simulink model "RUN_ME3_Helicopter_System_CDR"  (R2020b)
settings: Solver=VariableStepAuto  StartTime=0.0  StopTime=All_Sim_time  RelTol=1e-3
values from neighbouring files (symbols this model uses):
  All_Delay_betwn_actns = 28    [RUN_ME2_gui_to_tragectory.m]    (also in Workspace_CDR.mat = 30)
  All_Maneuver_smoothness = 16    [RUN_ME2_gui_to_tragectory.m]    (also in Workspace_CDR.mat = 28)
  K_CABLE = 3    [Coefficient_CDR.m]    (also in Workspace_CDR.mat)
  Kd_2 = PID_Elev_2.kd    [Coefficient_CDR.m]    (also in Workspace_CDR.mat = 79.7976366439)
  Kdp_2p = PID_Pitch_new_2pole.kd    [Coefficient_CDR.m]    (also in Workspace_CDR.mat = 43.0143282827)
  Kdt_2pole = PID_Travel_2pole.kd    [Coefficient_CDR.m]    (also in Workspace_CDR.mat = -1.1577862566)
  Ki_2 = PID_Elev_2.ki    [Coefficient_CDR.m]    (also in Workspace_CDR.mat = 88.2222308128)
  Kip_2p = PID_Pitch_new_2pole.ki    [Coefficient_CDR.m]    (also in Workspace_CDR.mat = 0)
  Kit_2pole = PID_Travel_2pole.ki    [Coefficient_CDR.m]    (also in Workspace_CDR.mat = -0.231061623642)
  Kp_2 = PID_Elev_2.kp    [Coefficient_CDR.m]    (also in Workspace_CDR.mat = 169.271716506)
  Kpp_2p = PID_Pitch_new_2pole.kp    [Coefficient_CDR.m]    (also in Workspace_CDR.mat = 367.16787657)
  Kpt_2pole = PID_Travel_2pole.kp    [Coefficient_CDR.m]    (also in Workspace_CDR.mat = -1.06540125736)
  Maneuver1_aggression = 20    [RUN_ME2_gui_to_tragectory.m]    (also in Workspace_CDR.mat)
  Maneuver2_aggression = 5    [RUN_ME2_gui_to_tragectory.m]    (also in Workspace_CDR.mat = 45)
  Maneuver3_aggression = 3    [RUN_ME2_gui_to_tragectory.m]    (also in Workspace_CDR.mat = 6.8)
  Maneuver4_aggression = 0.3    [RUN_ME2_gui_to_tragectory.m]    (also in Workspace_CDR.mat = 0.8)
  Maneuver5_aggression = 3.5    [RUN_ME2_gui_to_tragectory.m]    (also in Workspace_CDR.mat = 2.5)
libraries: simulink_extras x5, pid_lib x3, cstblocks x3
settings Model: Creator=justin  LastModifiedBy=liors

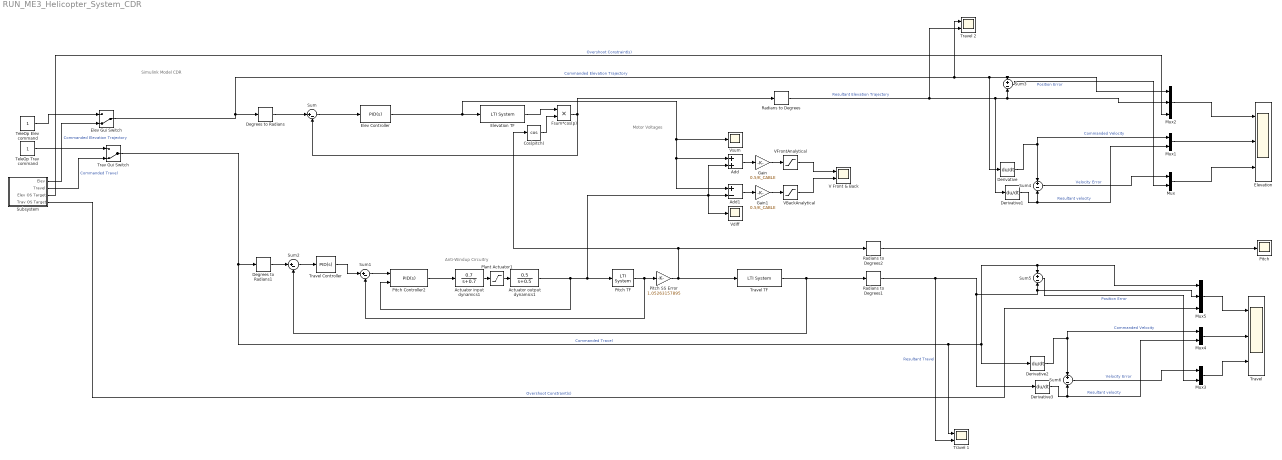
== system RUN_ME3_Helicopter_System_CDR ==
  note: Motor Voltages
  note: Anti-Windup Circuitry
  note: Simulink Model
      | CDR
  Actuator input dynamics1 : TransferFcn  Numerator=[0.7]  Denominator=[1 0.7]
  Actuator output dynamics1 : TransferFcn  Numerator=[0.5]  Denominator=[1 0.5]
  Add : Sum
  Add1 : Sum  Inputs=+-
  Cos(pitch) : Trigonometry  Operator=cos
  Degrees to Radians : simulink_extras/Transformations/Degrees to Radians
  Degrees to Radians1 : simulink_extras/Transformations/Degrees to Radians
  Derivative{,1..3} (4 alike) : Derivative
  Elev Controller : pid_lib/PID Controller  Controller=PID  Form=Parallel  TimeDomain=Continuous-time  UseExternalTs=off  SampleTime=-1  IntegratorMethod=Forward Euler  FilterMethod=Forward Euler  ControllerParametersSource=internal  P=Kp_2  I=Ki_2  D=Kd_2  UseFilter=on  N=100  TunerSelectOption=Transfer Function Based (PID Tuner App)  InitialConditionSource=internal  InitialConditionForIntegrator=0  InitialConditionForFilter=0  DifferentiatorICPrevScaledInput=0  ExternalReset=none  TrackingMode=off  Kt=150  LimitOutput=off  SatLimitsSource=internal  UpperSaturationLimit=inf  LowerSaturationLimit=0  LinearizeAsGain=on  AntiWindupMode=none  Kb=1  POutMin=[]  POutMax=[]  IOutMin=[]  IOutMax=[]  DOutMin=[]  DOutMax=[]  NOutMin=[]  NOutMax=[]  SumOutMin=[]  SumOutMax=[]  SaturationOutMin=[]  SaturationOutMax=[]  PParamMin=[]  PParamMax=[]  IParamMin=[]  IParamMax=[]  DParamMin=[]  DParamMax=[]  NParamMin=[]  NParamMax=[]  KbParamMin=[]  KbParamMax=[]  KtParamMin=[]  KtParamMax=[]  KbOutMin=[]  KbOutMax=[]  KtOutMin=[]  KtOutMax=[]  IntegratorOutMin=[]  IntegratorOutMax=[]  FilterOutMin=[]  FilterOutMax=[]  SumI1OutMin=[]  SumI1OutMax=[]  SumI2OutMin=[]  SumI2OutMax=[]  SumI3OutMin=[]  SumI3OutMax=[]  SumI4OutMin=[]  SumI4OutMax=[]  SumDOutMin=[]  SumDOutMax=[]  DifferentiatorOutMin=[]  DifferentiatorOutMax=[]  FilterDiffOutCoefMin=[]  FilterDiffOutCoefMax=[]  ReciprocalOutMin=[]  ReciprocalOutMax=[]  SumDenOutMin=[]  SumDenOutMax=[]  SumNumOutMin=[]  SumNumOutMax=[]  DivideOutMin=[]  DivideOutMax=[]  UdiffTsProdOutMin=[]  UdiffTsProdOutMax=[]  NTsProdOutMin=[]  NTsProdOutMax=[]  UintegralTsProdOutMin=[]  UintegralTsProdOutMax=[]  UngainTsProdOutMin=[]  UngainTsProdOutMax=[]  IntegratorContinuousStateAttributes=''  IntegratorStateMustResolveToSignalObject=off  IntegratorRTWStateStorageClass=Auto  FilterContinuousStateAttributes=''  FilterStateMustResolveToSignalObject=off  FilterRTWStateStorageClass=Auto  ParallelPVariant=InternalParameters  IdealPVariant=Disabled  IVariant=InternalParameters  DVariant=InternalParameters  IntegratorVariant=Continuous  SatVariant=Disabled  AWVariant=Passthrough  PCopyVariant=Disabled  TRVariant=Disabled  FdbkBlocksVariant=Forward  IdealPFdbkVariant=Disabled  SatFdbkVariant=Disabled  DerivativeFilterVariant=ContFilter  NVariant=InternalParameters  NCopyVariant=Disabled  FilterICVariant=InternalICsFilter  IntegratorICVariant=InternalICs  ExternalResetVariant=Disabled  TRSumVariant=Passthrough  SumFdbkVariant=Disabled  SumVariant=Sum_PID  TsampFilterVariant=InternalTs  TsampNgainVariant=Passthrough  TsampIntegralVariant=Passthrough  ExternalSaturationOutDataTypeStr=Inherit: Same as second input
  Elev Gui Switch : ManualSwitch  CurrentSetting=0
  Elevation : Scope  NumInputPorts=3
  Elevation TF : cstblocks/LTI System  sys=sys  IC=[-5.18]
  Fsum*cos(p) : Product
  Gain : Gain  Gain=0.5/K_CABLE
  Gain1 : Gain  Gain=0.5/K_CABLE
  Mux{,1,3..4} (4 alike) : Mux  Inputs=2
  Mux2 : Mux  Inputs=3
  Mux5 : Mux  Inputs=3
  "Pitch " : Scope
  Pitch Controller2 : pid_lib/PID Controller  Controller=PID  Form=Parallel  TimeDomain=Continuous-time  UseExternalTs=off  SampleTime=-1  IntegratorMethod=Forward Euler  FilterMethod=Forward Euler  ControllerParametersSource=internal  P=Kpp_2p  I=Kip_2p  D=Kdp_2p  UseFilter=on  N=100  TunerSelectOption=Transfer Function Based (PID Tuner App)  InitialConditionSource=internal  InitialConditionForIntegrator=0  InitialConditionForFilter=0  DifferentiatorICPrevScaledInput=0  ExternalReset=none  TrackingMode=on  Kt=75  LimitOutput=off  SatLimitsSource=internal  UpperSaturationLimit=2.94  LowerSaturationLimit=-2.94  LinearizeAsGain=on  AntiWindupMode=back-calculation  Kb=1000  POutMin=[]  POutMax=[]  IOutMin=[]  IOutMax=[]  DOutMin=[]  DOutMax=[]  NOutMin=[]  NOutMax=[]  SumOutMin=[]  SumOutMax=[]  SaturationOutMin=[]  SaturationOutMax=[]  PParamMin=[]  PParamMax=[]  IParamMin=[]  IParamMax=[]  DParamMin=[]  DParamMax=[]  NParamMin=[]  NParamMax=[]  KbParamMin=[]  KbParamMax=[]  KtParamMin=[]  KtParamMax=[]  KbOutMin=[]  KbOutMax=[]  KtOutMin=[]  KtOutMax=[]  IntegratorOutMin=[]  IntegratorOutMax=[]  FilterOutMin=[]  FilterOutMax=[]  SumI1OutMin=[]  SumI1OutMax=[]  SumI2OutMin=[]  SumI2OutMax=[]  SumI3OutMin=[]  SumI3OutMax=[]  SumI4OutMin=[]  SumI4OutMax=[]  SumDOutMin=[]  SumDOutMax=[]  DifferentiatorOutMin=[]  DifferentiatorOutMax=[]  FilterDiffOutCoefMin=[]  FilterDiffOutCoefMax=[]  ReciprocalOutMin=[]  ReciprocalOutMax=[]  SumDenOutMin=[]  SumDenOutMax=[]  SumNumOutMin=[]  SumNumOutMax=[]  DivideOutMin=[]  DivideOutMax=[]  UdiffTsProdOutMin=[]  UdiffTsProdOutMax=[]  NTsProdOutMin=[]  NTsProdOutMax=[]  UintegralTsProdOutMin=[]  UintegralTsProdOutMax=[]  UngainTsProdOutMin=[]  UngainTsProdOutMax=[]  IntegratorContinuousStateAttributes=''  IntegratorStateMustResolveToSignalObject=off  IntegratorRTWStateStorageClass=Auto  FilterContinuousStateAttributes=''  FilterStateMustResolveToSignalObject=off  FilterRTWStateStorageClass=Auto  ParallelPVariant=InternalParameters  IdealPVariant=Disabled  IVariant=InternalParameters  DVariant=InternalParameters  IntegratorVariant=Continuous  SatVariant=Disabled  AWVariant=Passthrough  PCopyVariant=Disabled  TRVariant=Enabled  FdbkBlocksVariant=Forward  IdealPFdbkVariant=Disabled  SatFdbkVariant=Disabled  DerivativeFilterVariant=ContFilter  NVariant=InternalParameters  NCopyVariant=Disabled  FilterICVariant=InternalICsFilter  IntegratorICVariant=InternalICs  ExternalResetVariant=Disabled  TRSumVariant=TrackingMode  SumFdbkVariant=Disabled  SumVariant=Sum_PID  TsampFilterVariant=InternalTs  TsampNgainVariant=Passthrough  TsampIntegralVariant=Passthrough  ExternalSaturationOutDataTypeStr=Inherit: Same as second input
  Pitch SS Error : Gain  Gain=1.05263157895
  Pitch TF : cstblocks/LTI System  sys=G_Pitch_new_2pole_1  IC=[]
  Plant Actuator1 : Saturate  UpperLimit=4  LowerLimit=-4
  Radians to Degrees : simulink_extras/Transformations/Radians to Degrees
  Radians to Degrees1 : simulink_extras/Transformations/Radians to Degrees
  Radians to Degrees2 : simulink_extras/Transformations/Radians to Degrees
  Subsystem : Subsystem
  Sum : Sum  Inputs=|+-
  Sum1 : Sum  Inputs=|+-
  Sum2 : Sum  Inputs=|+-
  Sum{3..6} (4 alike) : Sum  Inputs=+|-
  TeleOp Elev command : Constant
  TeleOp Trav command : Constant
  Trav Gui Switch : ManualSwitch  CurrentSetting=0
  Travel : Scope  NumInputPorts=3
  Travel 1 : Scope  NumInputPorts=2
  Travel 2 : Scope  NumInputPorts=2
  Travel Controller : pid_lib/PID Controller  Controller=PID  Form=Parallel  TimeDomain=Continuous-time  UseExternalTs=off  SampleTime=-1  IntegratorMethod=Forward Euler  FilterMethod=Forward Euler  ControllerParametersSource=internal  P=Kpt_2pole  I=Kit_2pole  D=Kdt_2pole  UseFilter=on  N=100  TunerSelectOption=Transfer Function Based (PID Tuner App)  InitialConditionSource=internal  InitialConditionForIntegrator=0  InitialConditionForFilter=0  DifferentiatorICPrevScaledInput=0  ExternalReset=none  TrackingMode=off  Kt=1  LimitOutput=off  SatLimitsSource=internal  UpperSaturationLimit=inf  LowerSaturationLimit=-inf  LinearizeAsGain=on  AntiWindupMode=none  Kb=1  POutMin=[]  POutMax=[]  IOutMin=[]  IOutMax=[]  DOutMin=[]  DOutMax=[]  NOutMin=[]  NOutMax=[]  SumOutMin=[]  SumOutMax=[]  SaturationOutMin=[]  SaturationOutMax=[]  PParamMin=[]  PParamMax=[]  IParamMin=[]  IParamMax=[]  DParamMin=[]  DParamMax=[]  NParamMin=[]  NParamMax=[]  KbParamMin=[]  KbParamMax=[]  KtParamMin=[]  KtParamMax=[]  KbOutMin=[]  KbOutMax=[]  KtOutMin=[]  KtOutMax=[]  IntegratorOutMin=[]  IntegratorOutMax=[]  FilterOutMin=[]  FilterOutMax=[]  SumI1OutMin=[]  SumI1OutMax=[]  SumI2OutMin=[]  SumI2OutMax=[]  SumI3OutMin=[]  SumI3OutMax=[]  SumI4OutMin=[]  SumI4OutMax=[]  SumDOutMin=[]  SumDOutMax=[]  DifferentiatorOutMin=[]  DifferentiatorOutMax=[]  FilterDiffOutCoefMin=[]  FilterDiffOutCoefMax=[]  ReciprocalOutMin=[]  ReciprocalOutMax=[]  SumDenOutMin=[]  SumDenOutMax=[]  SumNumOutMin=[]  SumNumOutMax=[]  DivideOutMin=[]  DivideOutMax=[]  UdiffTsProdOutMin=[]  UdiffTsProdOutMax=[]  NTsProdOutMin=[]  NTsProdOutMax=[]  UintegralTsProdOutMin=[]  UintegralTsProdOutMax=[]  UngainTsProdOutMin=[]  UngainTsProdOutMax=[]  IntegratorContinuousStateAttributes=''  IntegratorStateMustResolveToSignalObject=off  IntegratorRTWStateStorageClass=Auto  FilterContinuousStateAttributes=''  FilterStateMustResolveToSignalObject=off  FilterRTWStateStorageClass=Auto  ParallelPVariant=InternalParameters  IdealPVariant=Disabled  IVariant=InternalParameters  DVariant=InternalParameters  IntegratorVariant=Continuous  SatVariant=Disabled  AWVariant=Passthrough  PCopyVariant=Disabled  TRVariant=Disabled  FdbkBlocksVariant=Forward  IdealPFdbkVariant=Disabled  SatFdbkVariant=Disabled  DerivativeFilterVariant=ContFilter  NVariant=InternalParameters  NCopyVariant=Disabled  FilterICVariant=InternalICsFilter  IntegratorICVariant=InternalICs  ExternalResetVariant=Disabled  TRSumVariant=Passthrough  SumFdbkVariant=Disabled  SumVariant=Sum_PID  TsampFilterVariant=InternalTs  TsampNgainVariant=Passthrough  TsampIntegralVariant=Passthrough  ExternalSaturationOutDataTypeStr=Inherit: Same as second input
  Travel TF : cstblocks/LTI System  sys=G_Travel_new_2pole_1  IC=[]
  V Front & Back : Scope  NumInputPorts=2
  VBackAnalytical : Saturate  UpperLimit=22  LowerLimit=-22
  VFrontAnalytical : Saturate  UpperLimit=22  LowerLimit=-22
  Vdiff : Scope
  Vsum : Scope
  wires:
  Radians to Degrees/1 -> Travel 2/2, Mux2/2, Sum3/2, Derivative1/1  "Resultant Elevation Trajectory"
  Fsum*cos(p)/1 -> Sum/2, Radians to Degrees/1
  Travel TF/1 -> Sum2/2, Radians to Degrees1/1
  Degrees to Radians1/1 -> Sum2/1
  Radians to Degrees1/1 -> Travel 1/2, Derivative3/1, Mux5/2, Sum5/2  "Resultant Travel"
  Add/1 -> Gain/1
  Add1/1 -> Gain1/1
  Radians to Degrees2/1 -> "Pitch "/1
  Elev Gui Switch/1 -> Travel 2/1, Derivative/1, Sum3/1, Mux2/1, Degrees to Radians/1  "Commanded Elevation Trajectory"
  Gain/1 -> VFrontAnalytical/1
  VFrontAnalytical/1 -> V Front & Back/1
  Gain1/1 -> VBackAnalytical/1
  VBackAnalytical/1 -> V Front & Back/2
  Degrees to Radians/1 -> Sum/1
  Sum/1 -> Elev Controller/1
  Sum2/1 -> Travel Controller/1
  Cos(pitch)/1 -> Fsum*cos(p)/2
  Pitch TF/1 -> Pitch SS Error/1, Sum1/2
  Actuator input dynamics1/1 -> Plant Actuator1/1
  Plant Actuator1/1 -> Actuator output dynamics1/1
  Elev Controller/1 -> Add1/1, Add/1, Vsum/1, Elevation TF/1
  Actuator output dynamics1/1 -> Pitch Controller2/2, Vdiff/1, Add/2, Add1/2, Pitch TF/1
  Sum1/1 -> Pitch Controller2/1
  Travel Controller/1 -> Sum1/1
  Pitch SS Error/1 -> Cos(pitch)/1, Radians to Degrees2/1, Travel TF/1
  Pitch Controller2/1 -> Actuator input dynamics1/1
  Subsystem/3(Elev OS Target) -> Mux2/3  "Overshoot Constraint(s)"
  Subsystem/4(Trav OS Target) -> Mux5/3  "Overshoot Constraint(s)"
  Derivative/1 -> Mux1/1, Sum4/1  "Commanded Velocity"
  Derivative1/1 -> Sum4/2, Mux1/2  "Resultant velocity"
  Mux2/1 -> Elevation/1
  Mux1/1 -> Elevation/2
  Mux/1 -> Elevation/3
  Sum3/1 -> Mux/2  "Position Error"
  Sum4/1 -> Mux/1  "Velocity Error"
  Mux4/1 -> Travel/2
  Derivative2/1 -> Mux4/1, Sum6/1  "Commanded Velocity"
  Derivative3/1 -> Sum6/2, Mux4/2  "Resultant velocity"
  Sum5/1 -> Mux3/2  "Position Error"
  Mux5/1 -> Travel/1
  Mux3/1 -> Travel/3
  Sum6/1 -> Mux3/1  "Velocity Error"
  Trav Gui Switch/1 -> Travel 1/1, Mux5/1, Sum5/1, Derivative2/1, Degrees to Radians1/1  "Commanded Travel"
  TeleOp Trav command/1 -> Trav Gui Switch/1
  Subsystem/2(Travel) -> Trav Gui Switch/2  "Commanded Travel"
  Subsystem/1(Elev) -> Elev Gui Switch/2  "Commanded Elevation Trajectory"
  TeleOp Elev command/1 -> Elev Gui Switch/1
  Elevation TF/1 -> Fsum*cos(p)/1

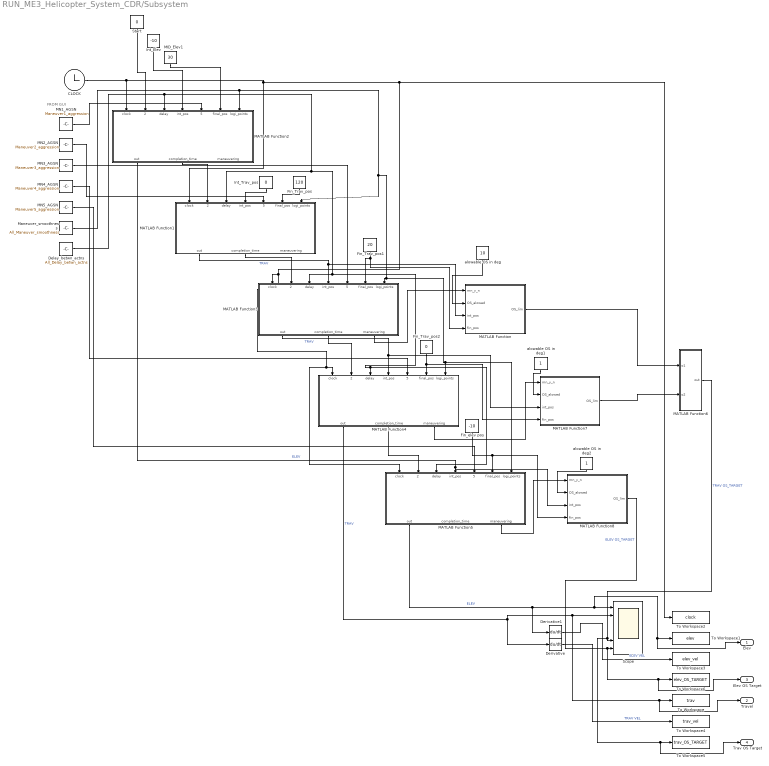
== system RUN_ME3_Helicopter_System_CDR/Subsystem ==
  note: FROM GUI
  CLOCK : Clock
  Delay_betwn_actns : Constant  Value=All_Delay_betwn_actns
  Derivative : Derivative
  Derivative1 : Derivative
  Fin_Trav_pos : Constant  Value=120
  Fin_Trav_pos1 : Constant  Value=20
  Fin_Trav_pos2 : Constant  Value=0
  Fin_elev pos : Constant  Value=-10
  Int_Elev : Constant  Value=-10
  Int_Trav_pos : Constant  Value=0
  MATLAB Function : MATLAB Function  TreatAsAtomicUnit=on
  MATLAB Function1 : MATLAB Function  TreatAsAtomicUnit=on
  MATLAB Function2 : MATLAB Function  TreatAsAtomicUnit=on
  MATLAB Function3 : MATLAB Function  TreatAsAtomicUnit=on
  MATLAB Function4 : MATLAB Function  TreatAsAtomicUnit=on
  MATLAB Function5 : MATLAB Function  TreatAsAtomicUnit=on
  MATLAB Function6 : MATLAB Function  TreatAsAtomicUnit=on
  MATLAB Function7 : MATLAB Function  TreatAsAtomicUnit=on
  MATLAB Function8 : MATLAB Function  TreatAsAtomicUnit=on
  MID_Elev1 : Constant  Value=30
  MN1_AGSN : Constant  Value=Maneuver1_aggression
  MN2_AGSN : Constant  Value=Maneuver2_aggression
  MN3_AGSN : Constant  Value=Maneuver3_aggression
  MN4_AGSN : Constant  Value=Maneuver4_aggression
  MN5_AGSN : Constant  Value=Maneuver5_aggression
  Maneuver_smoothness : Constant  Value=All_Maneuver_smoothness
  Scope : Scope  NumInputPorts=6
  Start : Constant  Value=0
  To Workspace : ToWorkspace  VariableName=trav  SaveFormat=Timeseries  SampleTime=-1
  To Workspace1 : ToWorkspace  VariableName=elev  SaveFormat=Timeseries  SampleTime=-1
  To Workspace2 : ToWorkspace  VariableName=clock  SaveFormat=Timeseries  SampleTime=-1
  To Workspace3 : ToWorkspace  VariableName=elev_vel  SaveFormat=Timeseries  SampleTime=-1
  To Workspace4 : ToWorkspace  VariableName=trav_vel  SaveFormat=Timeseries  SampleTime=-1
  To Workspace5 : ToWorkspace  VariableName=trav_OS_TARGET  SaveFormat=Timeseries  SampleTime=-1
  To Workspace6 : ToWorkspace  VariableName=elev_OS_TARGET  SaveFormat=Timeseries  SampleTime=-1
  alowable OS in deg : Constant  Value=10
  alowable OS in deg1 : Constant
  alowable OS in deg2 : Constant
  Elev : Outport
  Travel : Outport  Port=2
  Elev OS Target : Outport  Port=3
  Trav OS Target : Outport  Port=4
  wires:
  Derivative1/1 -> To Workspace3/1  "ELEV VEL"
  CLOCK/1 -> To Workspace2/1, MATLAB Function4/1(clock), MATLAB Function5/1(clock), MATLAB Function3/1(clock), MATLAB Function1/1(clock), MATLAB Function2/1(clock)
  MATLAB Function3/3(maneuvering) -> MATLAB Function/1(mn_y_n)
  Fin_elev pos/1 -> MATLAB Function8/4(fin_pos), MATLAB Function5/6(final_pos)
  MATLAB Function2/1(out) -> MATLAB Function8/3(int_pos), MATLAB Function5/4(int_pos)  "ELEV"
  Maneuver_smoothness/1 -> MATLAB Function4/7(logi_points), MATLAB Function5/7(logi_points), MATLAB Function3/7(logi_points), MATLAB Function1/7(logi_points), MATLAB Function2/7(logi_points)
  Int_Elev/1 -> MATLAB Function2/4(int_pos)
  Derivative/1 -> To Workspace4/1  "TRAV VEL"
  Start/1 -> MATLAB Function2/2(pev_mn_fin_time)
  MATLAB Function7/1(OS_lim) -> MATLAB Function6/2(o2)
  MN2_AGSN/1 -> MATLAB Function1/5(agressivness)
  MATLAB Function5/1(out) -> To Workspace1/1, Elev/1, Scope/1, Derivative1/1  "ELEV"
  MATLAB Function3/1(out) -> MATLAB Function7/3(int_pos), MATLAB Function4/4(int_pos)  "TRAV"
  alowable OS in deg1/1 -> MATLAB Function7/2(OS_alowed)
  Fin_Trav_pos1/1 -> MATLAB Function/4(fin_pos), MATLAB Function3/6(final_pos)
  MN5_AGSN/1 -> MATLAB Function5/5(agressivness)
  MATLAB Function1/1(out) -> MATLAB Function/3(int_pos), MATLAB Function3/4(int_pos)  "TRAV"
  Delay_betwn_actns/1 -> MATLAB Function5/3(delay), MATLAB Function4/3(delay), MATLAB Function3/3(delay), MATLAB Function1/3(delay), MATLAB Function2/3(delay)
  MN4_AGSN/1 -> MATLAB Function4/5(agressivness)
  MN1_AGSN/1 -> MATLAB Function2/5(agressivness)
  Int_Trav_pos/1 -> MATLAB Function1/4(int_pos)
  MATLAB Function3/2(completion_time) -> MATLAB Function4/2(pev_mn_fin_time)
  Fin_Trav_pos2/1 -> MATLAB Function7/4(fin_pos), MATLAB Function4/6(final_pos)
  alowable OS in deg/1 -> MATLAB Function/2(OS_alowed)
  MATLAB Function1/2(completion_time) -> MATLAB Function3/2(pev_mn_fin_time)
  MATLAB Function5/3(maneuvering) -> MATLAB Function8/1(mn_y_n)
  MATLAB Function2/2(completion_time) -> MATLAB Function1/2(pev_mn_fin_time)
  MN3_AGSN/1 -> MATLAB Function3/5(agressivness)
  Fin_Trav_pos/1 -> MATLAB Function1/6(final_pos)
  MID_Elev1/1 -> MATLAB Function2/6(final_pos)
  MATLAB Function4/1(out) -> Derivative/1, To Workspace/1, Travel/1, Scope/2  "TRAV"
  MATLAB Function6/1(out) -> Trav OS Target/1, To Workspace5/1, Scope/5  "TRAV OS_TARGET"
  MATLAB Function8/1(OS_lim) -> To Workspace6/1, Elev OS Target/1, Scope/6  "ELEV OS_TARGET"
  alowable OS in deg2/1 -> MATLAB Function8/2(OS_alowed)
  MATLAB Function/1(OS_lim) -> MATLAB Function6/1(o1)
  MATLAB Function4/3(maneuvering) -> MATLAB Function7/1(mn_y_n)
  MATLAB Function4/2(completion_time) -> MATLAB Function5/2(pev_mn_fin_time)

== matlab function RUN_ME3_Helicopter_System_CDR/Subsystem/MATLAB Function5 ==
  data: clock input; pev_mn_fin_time input; delay input; int_pos input; agressivness input; final_pos input; out output; completion_time output; logi_points input; maneuvering output
function [out,completion_time,maneuvering] =maneuver(clock,pev_mn_fin_time,delay,int_pos,agressivness,final_pos,logi_points)

if final_pos>int_pos
    direction=1
else
    direction=-1
end

slope=direction*agressivness
maneuvering=inf
mn_start_time=delay+pev_mn_fin_time
mn_completion_time=(final_pos-int_pos)/slope
completion_time=mn_completion_time+mn_start_time
coarsness=mn_completion_time/(logi_points+1)
mn_clock=clock-mn_start_time
coarse_clock=coarsness*floor(mn_clock/coarsness)
mn_clock2=clock+coarsness-mn_start_time
coarse_clock2=coarsness*floor(mn_clock2/coarsness)



if mn_clock<0
    out=int_pos
elseif clock<completion_time && mn_clock>=0
    adjust=mn_completion_time/18
    out1=((slope*mn_completion_time)/(1+exp((mn_completion_time/2-coarse_clock)/adjust)))    +int_pos
    out2=((slope*mn_completion_time)/(1+exp((mn_completion_time/2-coarse_clock2)/adjust)))    +int_pos
    sawtooth=mn_clock-coarse_clock
    new_slope=(out2-out1)/(coarsness)
    out=new_slope*sawtooth+out1
else
    out=final_pos
end

if mn_clock>=mn_completion_time/2
    maneuvering=1
end

if clock>=completion_time+delay+5/mn_completion_time
         maneuvering=inf
end
end

== matlab function RUN_ME3_Helicopter_System_CDR/Subsystem/MATLAB Function6 ==
  data: o1 input; out output; o2 input
function out= min(o1,o2)
out=min([o1,o2])
end

== matlab function RUN_ME3_Helicopter_System_CDR/Subsystem/MATLAB Function7 ==
  data: mn_y_n input; OS_lim output; OS_alowed input; int_pos input; fin_pos input
function OS_lim = OS(mn_y_n,OS_alowed,int_pos,fin_pos)
if fin_pos>int_pos
    direction=1
else
    direction=-1
end

OS_lim = mn_y_n*(fin_pos+OS_alowed*direction);
if OS_lim==-inf
   OS_lim=inf
end
end

== matlab function RUN_ME3_Helicopter_System_CDR/Subsystem/MATLAB Function8 ==
  data: mn_y_n input; OS_lim output; OS_alowed input; int_pos input; fin_pos input
function OS_lim = OS(mn_y_n,OS_alowed,int_pos,fin_pos)
if fin_pos>int_pos
    direction=1
else
    direction=-1
end

OS_lim = mn_y_n*(fin_pos+OS_alowed*direction);
if OS_lim==-inf
   OS_lim=inf
end
end

== matlab function RUN_ME3_Helicopter_System_CDR/Subsystem/MATLAB Function ==
  data: mn_y_n input; OS_lim output; OS_alowed input; int_pos input; fin_pos input
function OS_lim = OS(mn_y_n,OS_alowed,int_pos,fin_pos)
if fin_pos>int_pos
    direction=1
else
    direction=-1
end

OS_lim = mn_y_n*(fin_pos+OS_alowed*direction);
if OS_lim==-inf
   OS_lim=inf
end
end

== matlab function RUN_ME3_Helicopter_System_CDR/Subsystem/MATLAB Function1 ==
  data: clock input; pev_mn_fin_time input; delay input; int_pos input; agressivness input; final_pos input; out output; completion_time output; logi_points input; maneuvering output
function [out,completion_time,maneuvering] =maneuver(clock,pev_mn_fin_time,delay,int_pos,agressivness,final_pos,logi_points)

if final_pos>int_pos
    direction=1
else
    direction=-1
end

slope=direction*agressivness
maneuvering=inf
mn_start_time=delay+pev_mn_fin_time
mn_completion_time=(final_pos-int_pos)/slope
completion_time=mn_completion_time+mn_start_time
coarsness=mn_completion_time/(logi_points+1)
mn_clock=clock-mn_start_time
coarse_clock=coarsness*floor(mn_clock/coarsness)
mn_clock2=clock+coarsness-mn_start_time
coarse_clock2=coarsness*floor(mn_clock2/coarsness)



if mn_clock<0
    out=int_pos
elseif clock<completion_time && mn_clock>=0
adjust=mn_completion_time/20
    out1=((slope*mn_completion_time)/(1+exp((mn_completion_time/2-coarse_clock)/adjust)))    +int_pos
    out2=((slope*mn_completion_time)/(1+exp((mn_completion_time/2-coarse_clock2)/adjust)))    +int_pos
    sawtooth=mn_clock-coarse_clock
    new_slope=(out2-out1)/(coarsness)
    out=new_slope*sawtooth+out1-5.45e-3
else
    out=final_pos-5.45e-3
end

if mn_clock>=mn_completion_time/2
    maneuvering=1
end

if clock>=completion_time+delay+5/mn_completion_time
         maneuvering=inf
end

end

== matlab function RUN_ME3_Helicopter_System_CDR/Subsystem/MATLAB Function2 ==
  data: clock input; pev_mn_fin_time input; delay input; int_pos input; agressivness input; final_pos input; out output; completion_time output; logi_points input; maneuvering output
function [out,completion_time,maneuvering] =maneuver(clock,pev_mn_fin_time,delay,int_pos,agressivness,final_pos,logi_points)

if final_pos>int_pos
    direction=1
else
    direction=-1
end

slope=direction*agressivness
maneuvering=inf
mn_start_time=delay+pev_mn_fin_time
mn_completion_time=(final_pos-int_pos)/slope
completion_time=mn_completion_time+mn_start_time
coarsness=mn_completion_time/(logi_points+1)
mn_clock=clock-mn_start_time
coarse_clock=coarsness*floor(mn_clock/coarsness)
mn_clock2=clock+coarsness-mn_start_time
coarse_clock2=coarsness*floor(mn_clock2/coarsness)



if mn_clock<0
    out=int_pos
elseif clock<completion_time && mn_clock>=0
    adjust=mn_completion_time/18
    out1=((slope*mn_completion_time)/(1+exp((mn_completion_time/2-coarse_clock)/adjust)))    +int_pos
    out2=((slope*mn_completion_time)/(1+exp((mn_completion_time/2-coarse_clock2)/adjust)))    +int_pos
    sawtooth=mn_clock-coarse_clock
    new_slope=(out2-out1)/(coarsness)
    out=new_slope*sawtooth+out1
else
    out=final_pos
end

if mn_clock>=mn_completion_time/2
    maneuvering=1
end

if clock>=completion_time+delay+5/mn_completion_time
         maneuvering=inf
end
end

== matlab function RUN_ME3_Helicopter_System_CDR/Subsystem/MATLAB Function3 ==
  data: clock input; pev_mn_fin_time input; delay input; int_pos input; agressivness input; final_pos input; out output; completion_time output; logi_points input; maneuvering output
function [out,completion_time,maneuvering] =maneuver(clock,pev_mn_fin_time,delay,int_pos,agressivness,final_pos,logi_points)

if final_pos>int_pos
    direction=1
else
    direction=-1
end

slope=direction*agressivness
maneuvering=inf
mn_start_time=delay+pev_mn_fin_time
mn_completion_time=(final_pos-int_pos)/slope
completion_time=mn_completion_time+mn_start_time
coarsness=mn_completion_time/(logi_points+1)
mn_clock=clock-mn_start_time
coarse_clock=coarsness*floor(mn_clock/coarsness)
mn_clock2=clock+coarsness-mn_start_time
coarse_clock2=coarsness*floor(mn_clock2/coarsness)



if mn_clock<0
    out=int_pos
elseif clock<completion_time && mn_clock>=0
    adjust=mn_completion_time/18
    out1=((slope*mn_completion_time)/(1+exp((mn_completion_time/2-coarse_clock)/adjust)))    +int_pos
    out2=((slope*mn_completion_time)/(1+exp((mn_completion_time/2-coarse_clock2)/adjust)))    +int_pos
    sawtooth=mn_clock-coarse_clock
    new_slope=(out2-out1)/(coarsness)
    out=new_slope*sawtooth+out1
else
    out=final_pos
end

if mn_clock>=mn_completion_time/2
    maneuvering=1
end

if clock>=completion_time+delay+5/mn_completion_time
         maneuvering=inf
end
end

== matlab function RUN_ME3_Helicopter_System_CDR/Subsystem/MATLAB Function4 ==
  data: clock input; pev_mn_fin_time input; delay input; int_pos input; agressivness input; final_pos input; out output; completion_time output; logi_points input; maneuvering output
function [out,completion_time,maneuvering] =maneuver(clock,pev_mn_fin_time,delay,int_pos,agressivness,final_pos,logi_points)

if final_pos>int_pos
    direction=1
else
    direction=-1
end

slope=direction*agressivness
maneuvering=inf
mn_start_time=delay+pev_mn_fin_time
mn_completion_time=(final_pos-int_pos)/slope
completion_time=mn_completion_time+mn_start_time
coarsness=mn_completion_time/(logi_points+1)
mn_clock=clock-mn_start_time
coarse_clock=coarsness*floor(mn_clock/coarsness)
mn_clock2=clock+coarsness-mn_start_time
coarse_clock2=coarsness*floor(mn_clock2/coarsness)



if mn_clock<0
    out=int_pos
elseif clock<completion_time && mn_clock>=0
    adjust=mn_completion_time/18
    out1=((slope*mn_completion_time)/(1+exp((mn_completion_time/2-coarse_clock)/adjust)))    +int_pos
    out2=((slope*mn_completion_time)/(1+exp((mn_completion_time/2-coarse_clock2)/adjust)))    +int_pos
    sawtooth=mn_clock-coarse_clock
    new_slope=(out2-out1)/(coarsness)
    out=new_slope*sawtooth+out1
else
    out=final_pos
end

if mn_clock>=mn_completion_time/2
    maneuvering=1
end

if clock>=completion_time+delay+5/mn_completion_time
         maneuvering=inf
end
end
